simulink model "simuladorControlCuatrirrotor"  (Simulink 8.0)
settings: Solver=ode45  StartTime=0.0  StopTime=100  FixedStep=0.06  MaxStep=Ts  RelTol=1e-3
values from neighbouring files (symbols this model uses):
  radio = 0.1    [simulaControl.m]
  ruta = [0,0;ruta]    [pintascdata.m]    (also in pintascdata_tb2.m; simulaControl.m = [12 12;12 12])
undefined symbols (not defined in the file or in its folder): DiscIntNeverNeededParam, Ts
libraries: simulink x6, slident x2
settings Model: Creator=xblasco  LastModifiedBy=Elisa
settings DataIOCC: SignalLoggingSaveFormat=ModelDataLogs
settings DebuggingCC: FcnCallInpInsideContextMsg=UseLocalSettings  StrictBusMsg=Warning
settings GRTTargetCC: CombineOutputUpdateFcns=off  GRTInterface=on

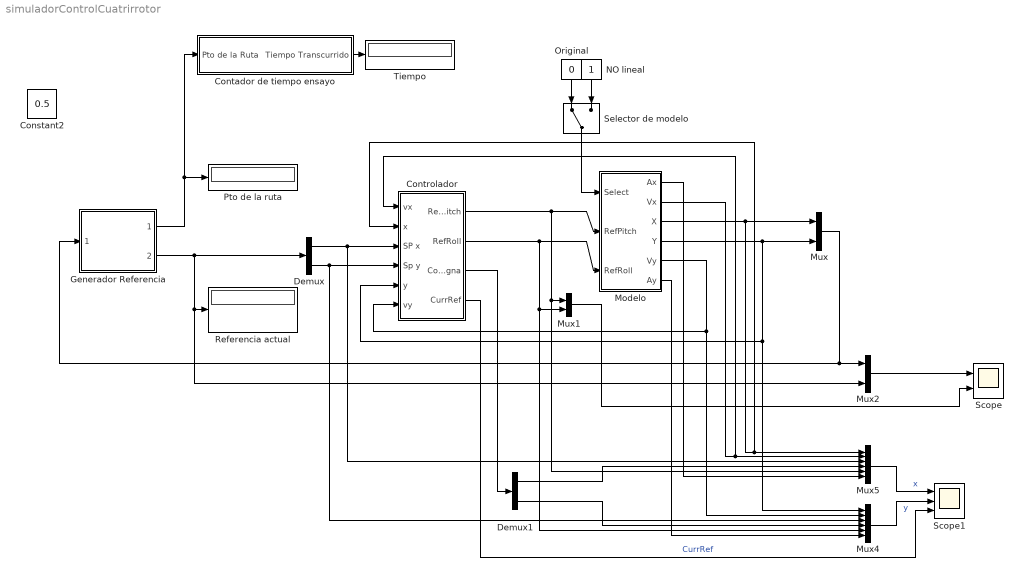
== system simuladorControlCuatrirrotor ==
  Contador de tiempo ensayo : Subsystem
  Controlador : Subsystem
  Demux : Demux  Outputs=2
  Demux1 : Demux  Outputs=2
  Generador Referencia : Subsystem
  Modelo : Subsystem
  Mux : Mux  Inputs=2
  Mux1 : Mux  Inputs=2
  Mux2 : Mux  Inputs=2
  Mux4 : Mux  Inputs=6
  Mux5 : Mux  Inputs=6
  NO lineal : Constant
  Original : Constant  Value=0
  Pto de la ruta : Display
  Referencia actual : Display
  Scope : Scope  NumInputPorts=2
      settings: YMin=-5~-1  YMax=15~1  SaveName=scdata  SampleInput=on  SampleTime=0.06
  Scope1 : Scope  NumInputPorts=3
      settings: YMin=-5~-1~-5  YMax=15~1~5  SaveName=scVar  SampleInput=on  SampleTime=0.06
  Selector de modelo : ManualSwitch
  Tiempo : Display
  Constant2 : Constant  IOType=siggen  Value=0.5
  wires:
  Generador Referencia/2(Siguiente pos) -> Mux2/2, Referencia actual/1, Demux/1
  Generador Referencia/1(Pto de la ruta) -> Pto de la ruta/1, Contador de tiempo ensayo/1(Pto de la Ruta)
  Mux/1 -> Mux2/1, Generador Referencia/1(Posicion  actual)
  Controlador/2(RefRoll) -> Mux4/5, Mux1/2, Modelo/3(RefRoll)
  Controlador/1(RefPitch) -> Mux5/5, Mux1/1, Modelo/2(RefPitch)
  Mux1/1 -> Scope/2
  Mux2/1 -> Scope/1
  Demux/1 -> Controlador/3(SP x), Mux5/3
  Demux/2 -> Controlador/4(Sp y), Mux4/3
  Contador de tiempo ensayo/1(Tiempo Transcurrido) -> Tiempo/1
  Mux4/1 -> Scope1/2  "y"
  Mux5/1 -> Scope1/1  "x"
  Controlador/3(Consigna) -> Demux1/1
  Demux1/1 -> Mux5/4
  Demux1/2 -> Mux4/4
  Controlador/4(CurrRef) -> Scope1/3  "CurrRef"
  Modelo/5(Vy) -> Controlador/6(vy), Mux4/2
  Modelo/4(Y) -> Mux/2, Controlador/5(y), Mux4/1
  Modelo/2(Vx) -> Controlador/1(vx), Mux5/2
  Modelo/3(X) -> Controlador/2(x), Mux5/1, Mux/1
  Selector de modelo/1 -> Modelo/1(Select)
  Original/1 -> Selector de modelo/1
  NO lineal/1 -> Selector de modelo/2
  Modelo/1(Ax) -> Mux5/6
  Modelo/6(Ay) -> Mux4/6

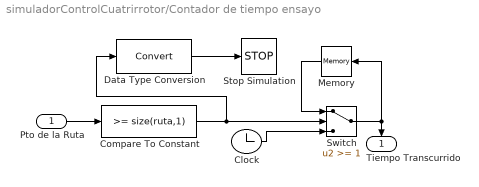
== system simuladorControlCuatrirrotor/Contador de tiempo ensayo ==
  Pto de la Ruta : Inport
  Clock : Clock
  Compare To Constant : simulink/Logic and Bit Operations/Compare To Constant  relop=>=  const=size(ruta,1)  OutDataTypeStr=uint8
  Data Type Conversion : DataTypeConversion
  Memory : Memory
  Stop Simulation : Stop
  Switch : Switch  Threshold=1
  Tiempo Transcurrido : Outport
  wires:
  Clock/1 -> Switch/3
  Compare To Constant/1 -> Switch/2, Data Type Conversion/1
  Switch/1 -> Memory/1, Tiempo Transcurrido/1
  Memory/1 -> Switch/1
  Data Type Conversion/1 -> Stop Simulation/1
  Pto de la Ruta/1 -> Compare To Constant/1

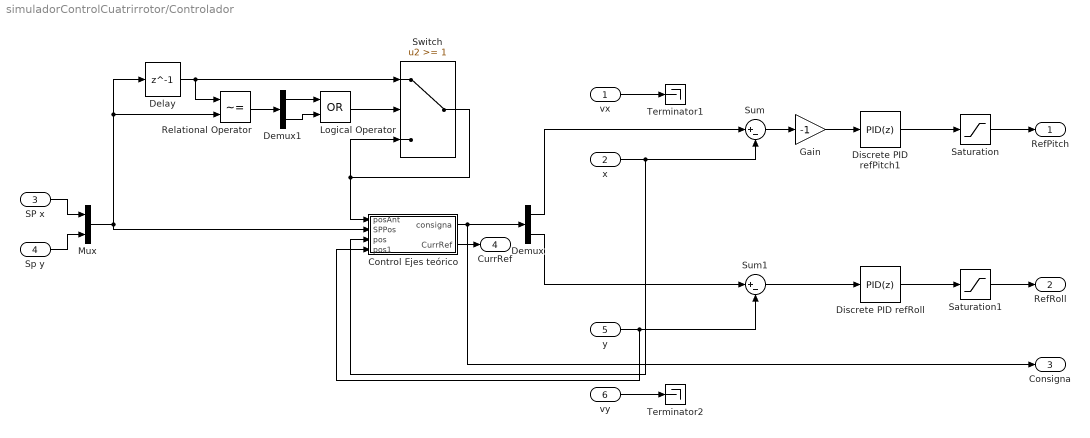
== system simuladorControlCuatrirrotor/Controlador ==
  vx : Inport
  x : Inport  Port=2
  SP x : Inport  Port=3
  Sp y : Inport  Port=4
  y : Inport  Port=5
  vy : Inport  Port=6
  Control Ejes teórico : Subsystem
  Delay : Delay  DelayLength=1  InitialCondition=0  SampleTime=Ts
  Demux : Demux  Outputs=2
  Demux1 : Demux  Outputs=2
  Discrete PID refPitch1 : simulink/Continuous/PID Controller  Controller=PID  TimeDomain=Discrete-time  SampleTime=Ts  IntegratorMethod=Forward Euler  FilterMethod=Forward Euler  Form=Parallel  P=0.65  I=0  D=0.5  N=15  InitialConditionSource=internal  InitialConditionForIntegrator=0  InitialConditionForFilter=0  ExternalReset=none  LimitOutput=off  UpperSaturationLimit=inf  LowerSaturationLimit=-inf  LinearizeAsGain=off  AntiWindupMode=none  Kb=1  TrackingMode=off  Kt=1  PParamMin=[]  PParamMax=[]  IParamMin=[]  IParamMax=[]  DParamMin=[]  DParamMax=[]  NParamMin=[]  NParamMax=[]  KbParamMin=[]  KbParamMax=[]  KtParamMin=[]  KtParamMax=[]  POutMin=[]  POutMax=[]  IOutMin=[]  IOutMax=[]  DOutMin=[]  DOutMax=[]  NOutMin=[]  NOutMax=[]  KbOutMin=[]  KbOutMax=[]  KtOutMin=[]  KtOutMax=[]  IntegratorOutMin=[]  IntegratorOutMax=[]  FilterOutMin=[]  FilterOutMax=[]  SumOutMin=[]  SumOutMax=[]  SumI1OutMin=[]  SumI1OutMax=[]  SumI2OutMin=[]  SumI2OutMax=[]  SumI3OutMin=[]  SumI3OutMax=[]  SumDOutMin=[]  SumDOutMax=[]  SaturationOutMin=[]  SaturationOutMax=[]  IntegratorContinuousStateAttributes=''  IntegratorStateMustResolveToSignalObject=off  IntegratorRTWStateStorageClass=Auto  FilterContinuousStateAttributes=''  FilterStateMustResolveToSignalObject=off  FilterRTWStateStorageClass=Auto
  Discrete PID refRoll : simulink/Continuous/PID Controller  Controller=PID  TimeDomain=Discrete-time  SampleTime=Ts  IntegratorMethod=Forward Euler  FilterMethod=Forward Euler  Form=Parallel  P=0.95  I=0.002  D=0.5  N=10  InitialConditionSource=internal  InitialConditionForIntegrator=0  InitialConditionForFilter=0  ExternalReset=none  LimitOutput=off  UpperSaturationLimit=inf  LowerSaturationLimit=-inf  LinearizeAsGain=off  AntiWindupMode=none  Kb=1  TrackingMode=off  Kt=1  PParamMin=[]  PParamMax=[]  IParamMin=[]  IParamMax=[]  DParamMin=[]  DParamMax=[]  NParamMin=[]  NParamMax=[]  KbParamMin=[]  KbParamMax=[]  KtParamMin=[]  KtParamMax=[]  POutMin=[]  POutMax=[]  IOutMin=[]  IOutMax=[]  DOutMin=[]  DOutMax=[]  NOutMin=[]  NOutMax=[]  KbOutMin=[]  KbOutMax=[]  KtOutMin=[]  KtOutMax=[]  IntegratorOutMin=[]  IntegratorOutMax=[]  FilterOutMin=[]  FilterOutMax=[]  SumOutMin=[]  SumOutMax=[]  SumI1OutMin=[]  SumI1OutMax=[]  SumI2OutMin=[]  SumI2OutMax=[]  SumI3OutMin=[]  SumI3OutMax=[]  SumDOutMin=[]  SumDOutMax=[]  SaturationOutMin=[]  SaturationOutMax=[]  IntegratorContinuousStateAttributes=''  IntegratorStateMustResolveToSignalObject=off  IntegratorRTWStateStorageClass=Auto  FilterContinuousStateAttributes=''  FilterStateMustResolveToSignalObject=off  FilterRTWStateStorageClass=Auto
  Gain : Gain  Gain=-1  SampleTime=Ts
  Logical Operator : Logic  Operator=OR  AllPortsSameDT=off  OutDataTypeStr=boolean  SampleTime=Ts
  Mux : Mux  Inputs=2
  Relational Operator : RelationalOperator  Operator=~=  OutDataTypeStr=boolean
  Saturation : Saturate  SampleTime=Ts
  Saturation1 : Saturate  SampleTime=Ts
  Sum : Sum  Inputs=|+-
  Sum1 : Sum  Inputs=|+-
  Switch : Switch  Threshold=1  SampleTime=Ts
  Terminator1 : Terminator
  Terminator2 : Terminator
  RefPitch : Outport
  RefRoll : Outport  Port=2
  Consigna : Outport  Port=3
  CurrRef : Outport  Port=4
  wires:
  Saturation/1 -> RefPitch/1
  x/1 -> Control Ejes teórico/3(pos), Sum/2
  vx/1 -> Terminator1/1
  vy/1 -> Terminator2/1
  Sum/1 -> Gain/1
  Gain/1 -> Discrete PID refPitch1/1
  Saturation1/1 -> RefRoll/1
  Discrete PID refRoll/1 -> Saturation1/1
  Discrete PID refPitch1/1 -> Saturation/1
  SP x/1 -> Mux/1
  Sp y/1 -> Mux/2
  Mux/1 -> Control Ejes teórico/2(SPPos), Delay/1, Relational Operator/2
  Control Ejes teórico/1(consigna) -> Consigna/1, Demux/1
  y/1 -> Control Ejes teórico/4(pos1), Sum1/2
  Sum1/1 -> Discrete PID refRoll/1
  Demux/2 -> Sum1/1
  Demux/1 -> Sum/1
  Relational Operator/1 -> Demux1/1
  Delay/1 -> Relational Operator/1, Switch/1
  Switch/1 -> Switch/3, Control Ejes teórico/1(posAnt)
  Demux1/1 -> Logical Operator/1
  Demux1/2 -> Logical Operator/2
  Logical Operator/1 -> Switch/2
  Control Ejes teórico/2(CurrRef) -> CurrRef/1

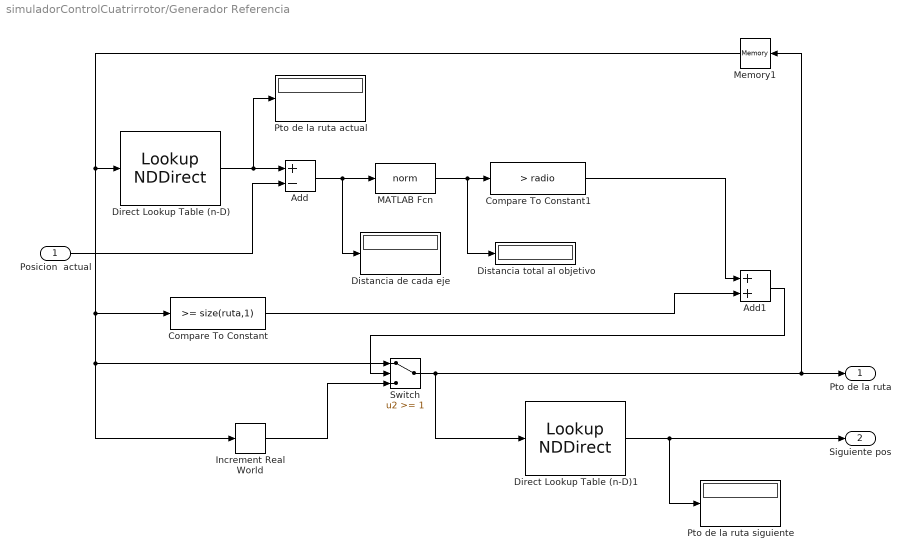
== system simuladorControlCuatrirrotor/Generador Referencia ==
  Posicion  actual : Inport
  Add : Sum  Inputs=+-
  Add1 : Sum
  Compare To Constant : simulink/Logic and Bit Operations/Compare To Constant  relop=>=  const=size(ruta,1)  OutDataTypeStr=uint8
  Compare To Constant1 : simulink/Logic and Bit Operations/Compare To Constant  relop=>  const=radio  OutDataTypeStr=uint8
  Direct Lookup Table (n-D) : LookupNDDirect  InputsSelectThisObjectFromTable=Column  Table=ruta'
  Direct Lookup Table (n-D)1 : LookupNDDirect  InputsSelectThisObjectFromTable=Column  Table=ruta'
  Distancia de cada eje : Display
  Distancia total al objetivo : Display
  Increment Real World : simulink/Additional Math & Discrete/Additional Math: Increment - Decrement/Increment Real World
  MATLAB Fcn : MATLABFcn  MATLABFcn=norm  Output1D=off
  Memory1 : Memory
  Pto de la ruta actual : Display
  Pto de la ruta siguiente : Display
  Switch : Switch  Threshold=1
  Pto de la ruta : Outport
  Siguiente pos : Outport  Port=2
  wires:
  Direct Lookup Table (n-D)/1 -> Pto de la ruta actual/1, Add/1
  Add/1 -> Distancia de cada eje/1, MATLAB Fcn/1
  Increment Real World/1 -> Switch/3
  Switch/1 -> Memory1/1, Pto de la ruta/1, Direct Lookup Table (n-D)1/1
  Posicion  actual/1 -> Add/2
  Direct Lookup Table (n-D)1/1 -> Siguiente pos/1, Pto de la ruta siguiente/1
  MATLAB Fcn/1 -> Compare To Constant1/1, Distancia total al objetivo/1
  Compare To Constant1/1 -> Add1/1
  Compare To Constant/1 -> Add1/2
  Add1/1 -> Switch/2
  Memory1/1 -> Direct Lookup Table (n-D)/1, Switch/1, Increment Real World/1, Compare To Constant/1

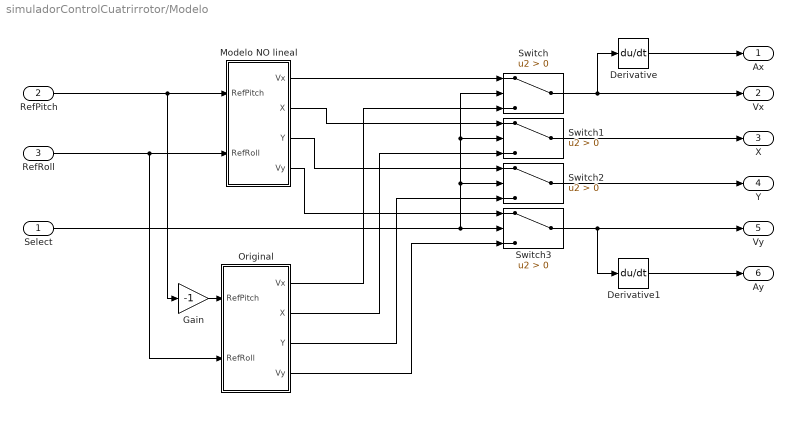
== system simuladorControlCuatrirrotor/Modelo ==
  Select : Inport
  RefPitch : Inport  Port=2
  RefRoll : Inport  Port=3
  " Modelo NO lineal" : Subsystem
  " Original" : Subsystem
  Derivative : Derivative
  Derivative1 : Derivative
  Gain : Gain  Gain=-1
  Switch{,1..3} (4 alike) : Switch  Criteria=u2 > Threshold
  Ax : Outport
  Vx : Outport  Port=2
  X : Outport  Port=3
  Y : Outport  Port=4
  Vy : Outport  Port=5
  Ay : Outport  Port=6
  wires:
  " Modelo NO lineal"/1(Vx) -> Switch/1
  RefPitch/1 -> Gain/1, " Modelo NO lineal"/1(RefPitch)
  RefRoll/1 -> " Original"/2(RefRoll), " Modelo NO lineal"/2(RefRoll)
  " Original"/1(Vx) -> Switch/3
  Select/1 -> Switch3/2, Switch2/2, Switch1/2, Switch/2
  Switch/1 -> Vx/1, Derivative/1
  Switch1/1 -> X/1
  Switch2/1 -> Y/1
  Switch3/1 -> Vy/1, Derivative1/1
  " Original"/2(X) -> Switch1/3
  " Original"/3(Y) -> Switch2/3
  " Original"/4(Vy) -> Switch3/3
  " Modelo NO lineal"/2(X) -> Switch1/1
  " Modelo NO lineal"/3(Y) -> Switch2/1
  " Modelo NO lineal"/4(Vy) -> Switch3/1
  Gain/1 -> " Original"/1(RefPitch)
  Derivative/1 -> Ax/1
  Derivative1/1 -> Ay/1

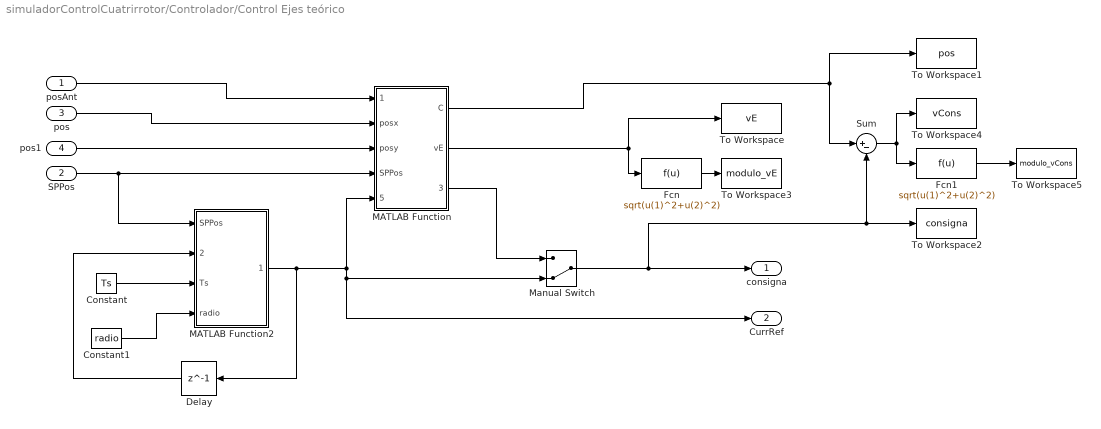
== system simuladorControlCuatrirrotor/Controlador/Control Ejes teórico ==
  posAnt : Inport
  SPPos : Inport  Port=2
  pos : Inport  Port=3
  pos1 : Inport  Port=4
  Constant : Constant  Value=Ts
  Constant1 : Constant  Value=radio
  Delay : Delay  DelayLength=1  InitialCondition=0  SampleTime=Ts
  Fcn : Fcn  Expr=sqrt(u(1)^2+u(2)^2)
  Fcn1 : Fcn  Expr=sqrt(u(1)^2+u(2)^2)
  MATLAB Function : MATLAB Function  TreatAsAtomicUnit=on
  MATLAB Function2 : MATLAB Function  TreatAsAtomicUnit=on  SystemSampleTime=Ts
  Manual Switch : ManualSwitch  CurrentSetting=0
  Sum : Sum  Inputs=|+-
  To Workspace : ToWorkspace  VariableName=vE  SampleTime=-1
  To Workspace1 : ToWorkspace  VariableName=pos  SampleTime=-1
  To Workspace2 : ToWorkspace  VariableName=consigna  SampleTime=-1
  To Workspace3 : ToWorkspace  VariableName=modulo_vE  SampleTime=-1  SaveFormat=Structure With Time
  To Workspace4 : ToWorkspace  VariableName=vCons  SampleTime=-1
  To Workspace5 : ToWorkspace  VariableName=modulo_vCons  SampleTime=-1  SaveFormat=Structure With Time
  consigna : Outport
  CurrRef : Outport  Port=2
  wires:
  SPPos/1 -> MATLAB Function/4(SPPos), MATLAB Function2/1(SPPos)
  Constant/1 -> MATLAB Function2/3(Ts)
  Constant1/1 -> MATLAB Function2/4(radio)
  posAnt/1 -> MATLAB Function/1(posAnt)
  pos/1 -> MATLAB Function/2(posx)
  Delay/1 -> MATLAB Function2/2(LastRef)
  MATLAB Function2/1(CurrRef) -> MATLAB Function/5(CurrRef), Manual Switch/2, CurrRef/1, Delay/1
  MATLAB Function/3(consigna) -> Manual Switch/1
  Manual Switch/1 -> To Workspace2/1, Sum/2, consigna/1
  pos1/1 -> MATLAB Function/3(posy)
  MATLAB Function/2(vE) -> To Workspace/1, Fcn/1
  MATLAB Function/1(C) -> Sum/1, To Workspace1/1
  Fcn/1 -> To Workspace3/1
  Sum/1 -> Fcn1/1, To Workspace4/1
  Fcn1/1 -> To Workspace5/1

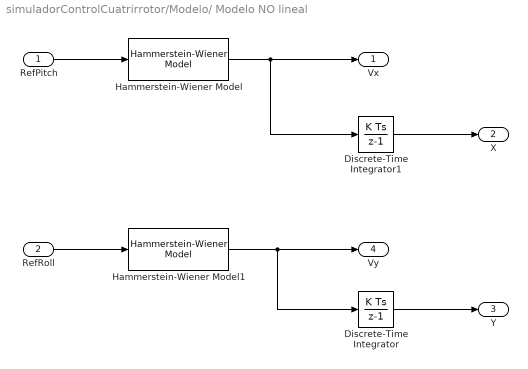
== system simuladorControlCuatrirrotor/Modelo/ Modelo NO lineal ==
  RefPitch : Inport  PortDimensions=1  SampleTime=0.06
  RefRoll : Inport  Port=2  PortDimensions=1  SampleTime=0.06
  Discrete-Time Integrator : DiscreteIntegrator  SampleTime=Ts  ICPrevOutput=DiscIntNeverNeededParam  ICPrevScaledInput=DiscIntNeverNeededParam
  Discrete-Time Integrator1 : DiscreteIntegrator  SampleTime=Ts  ICPrevOutput=DiscIntNeverNeededParam  ICPrevScaledInput=DiscIntNeverNeededParam
  Hammerstein-Wiener Model : slident/Hammerstein-Wiener Model  sys=vx123_nlhw113_pic2  IC=Zero  X0i=0
  Hammerstein-Wiener Model1 : slident/Hammerstein-Wiener Model  sys=vy123_nlhw111  IC=Zero  X0i=0
  Vx : Outport
  X : Outport  Port=2
  Y : Outport  Port=3
  Vy : Outport  Port=4
  wires:
  Hammerstein-Wiener Model1/1 -> Discrete-Time Integrator/1, Vy/1
  Hammerstein-Wiener Model/1 -> Discrete-Time Integrator1/1, Vx/1
  RefRoll/1 -> Hammerstein-Wiener Model1/1
  RefPitch/1 -> Hammerstein-Wiener Model/1
  Discrete-Time Integrator/1 -> Y/1
  Discrete-Time Integrator1/1 -> X/1

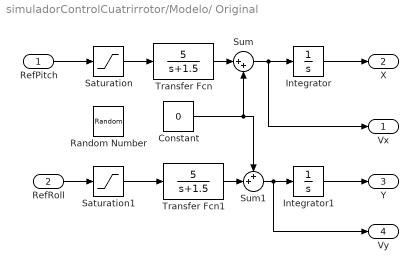
== system simuladorControlCuatrirrotor/Modelo/ Original ==
  RefPitch : Inport  PortDimensions=1  SampleTime=0.06
  RefRoll : Inport  Port=2  PortDimensions=1  SampleTime=0.06
  Constant : Constant  Value=0
  Integrator : Integrator
  Integrator1 : Integrator
  Random Number : RandomNumber  Variance=0.3  SampleTime=0.06
  Saturation : Saturate  UpperLimit=1  LowerLimit=-1
  Saturation1 : Saturate  UpperLimit=1  LowerLimit=-1
  Sum : Sum  Inputs=|++
  Sum1 : Sum  Inputs=++|
  Transfer Fcn : TransferFcn  Numerator=[5]  Denominator=[1 1.5]
  Transfer Fcn1 : TransferFcn  Numerator=[5]  Denominator=[1 1.5]
  Vx : Outport
  X : Outport  Port=2
  Y : Outport  Port=3
  Vy : Outport  Port=4
  wires:
  RefPitch/1 -> Saturation/1
  RefRoll/1 -> Saturation1/1
  Integrator/1 -> X/1
  Integrator1/1 -> Y/1
  Saturation/1 -> Transfer Fcn/1
  Saturation1/1 -> Transfer Fcn1/1
  Transfer Fcn/1 -> Sum/1
  Sum/1 -> Integrator/1, Vx/1
  Transfer Fcn1/1 -> Sum1/2
  Sum1/1 -> Integrator1/1, Vy/1
  Constant/1 -> Sum1/1, Sum/2

== matlab function Controlador/Control Ejes teórico/MATLAB Function ==
  data: C output double; vE output double; posAnt input double; posx input double; posy input double; SPPos input double; CurrRef input double; consigna output double
function [C,vE,consigna] = CalcRef(posAnt,posx,posy,SPPos,CurrRef)

A=posAnt;
B=SPPos;
C=[posx;posy]; %construimos vector posicion

% creamos vector director de la recta AB (recta r)
Vr = B-A;

% iniciamos vector Vs
Vs = Vr;

% creamos vector perpendicular a Vr
Vs(1,1) = -Vr(2,1);
Vs(2,1) = Vr(1,1);

% creamos matriz de vectores directores
MatrA = [Vr,-Vs];

% creamos matriz de valores independientes
MatrB = C-A;

% calculamos los valores de las K's de cada recta
K = inv(MatrA)*MatrB;

% sacamos el punto D intereseccion de las rectas
D = A + K(1,1)*Vr;

vE = D-C;

consigna = CurrRef + vE*20;
end

== matlab function Controlador/Control Ejes teórico/MATLAB Function2 ==
  data: CurrRef output double size=2; SPPos input double; LastRef input double; Ts input double; radio input double
function CurrRef = CalcRef(SPPos,LastRef,Ts,radio)
% Este bloque es un control de ambas velocidades a título teórico para
% definir las consignas a seguir según una velocidad máxima teórica
% constante obtenida experimentalmente en los modelos. No ayuda gran cosa a
% corregir las imprecisiones en la trayectoria y el desincronismo de los
% ejes se refleja igualmente con una diferencia notable desde el arranque.

maxVx = 1.5; % (-)Pitch
maxVy = 0.5; % Roll

DistXY =SPPos-LastRef;

if (norm(DistXY)<(0.5*radio)) % (0.5*radio)
    CurrRef = LastRef;
else
    minTx = abs (DistXY(1))/maxVx;
    minTy = abs (DistXY(2))/maxVy;
    
    minT = max (minTx,minTy);
    
    if minT<Ts
        CurrRef = SPPos;
    else
        CurrRef = LastRef + (Ts/minT)*DistXY;
    end
end
